simulink model "RC3_ECM"  (R2025a)
settings: Solver=VariableStepAuto  StartTime=0.0  StopTime=length(Current)  RelTol=1e-3
values from neighbouring files (symbols this model uses):
  C1_est = [C1_est(1); C1_est]    [RC3_Parameter_Extract.m]
  C2_est = [C2_est(1); C2_est]    [RC3_Parameter_Extract.m]
  C3_est = [C3_est(1); C3_est]    [RC3_Parameter_Extract.m]
  OCV_fit = flipud(OCV_fit)    [RC3_Parameter_Extract.m]    (also in RC3_Parameter_Tuning.m)
  R0_est = [R0_est(1); R0_est]    [RC3_Parameter_Extract.m]
  R1_est = [R1_est(1); R1_est]    [RC3_Parameter_Extract.m]    (also in RC3_Parameter_Tuning.m = R1_est/10)
  R2_est = [R0_est(1); R2_est]    [RC3_Parameter_Extract.m]
  R3_est = [R3_est(1); R3_est]    [RC3_Parameter_Extract.m]
  SOC_OCV = [0:0.05:1]'    [RC3_Parameter_Extract.m]    (also in RC3_Parameter_Tuning.m)
  SOC_RC = [0:0.05:1]'    [RC3_Parameter_Extract.m]    (also in RC3_Parameter_Tuning.m = [0.05:0.05:1]')
undefined symbols (not defined in the file or in its folder): OCV, Ri, SOC
settings Model: Creator=Administrator  LastModifiedBy=Administrator

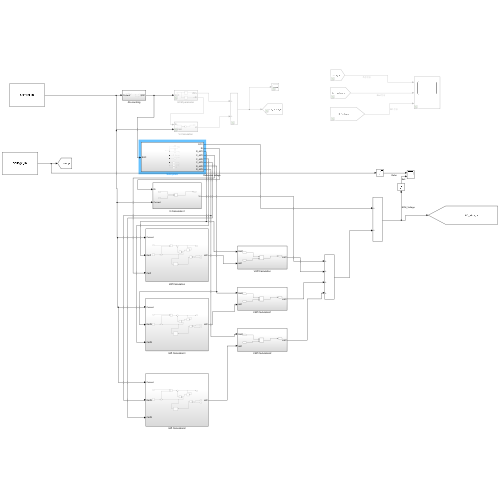
[thumbnail: Simulink's stored preview of the top-level diagram]
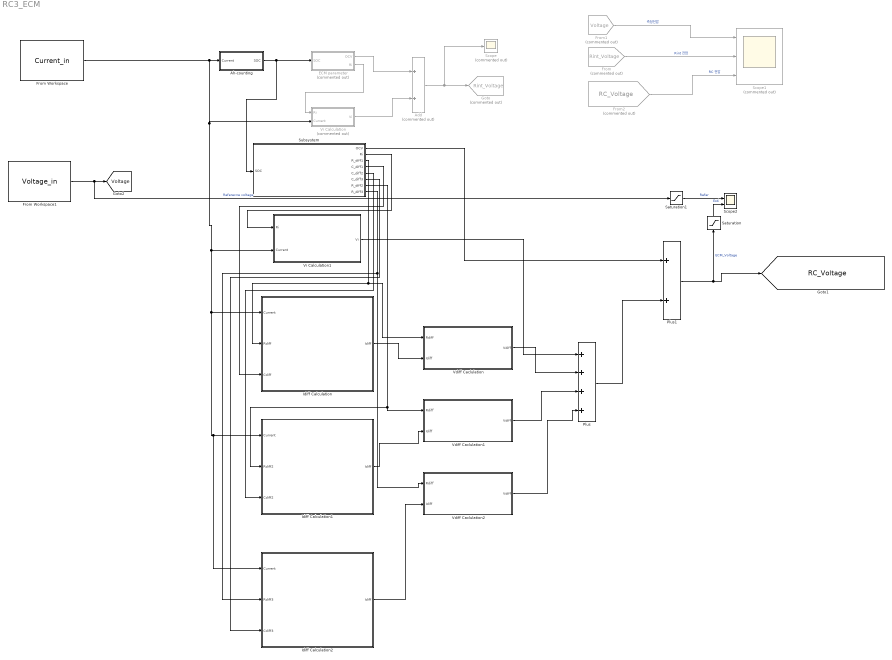
== system RC3_ECM ==
  Add : Sum  Commented=on
  Ah-counting : Subsystem
  ECM parameter : Subsystem  Commented=on
  From : From  Commented=on  GotoTag=Rint_Voltage  TagVisibility=global
  From Workspace : FromWorkspace  VariableName=Current_in  OutDataTypeStr=double  SampleTime=1
  From Workspace1 : FromWorkspace  VariableName=Voltage_in  OutDataTypeStr=double  SampleTime=1
  From1 : From  Commented=on  GotoTag=Voltage  TagVisibility=global
  From2 : From  Commented=on  GotoTag=RC_Voltage  TagVisibility=global
  Goto : Goto  Commented=on  GotoTag=Rint_Voltage  TagVisibility=global
  Idiff Calculation : Subsystem
  Idiff Calculation1 : Subsystem
  Idiff Calculation2 : Subsystem
  Plus : Sum  Inputs=++++
  Plus1 : Sum
  Saturation : Saturate  UpperLimit=4.5  LowerLimit=2.0
  Saturation1 : Saturate  UpperLimit=4.5  LowerLimit=2.0
  Scope : Scope  Commented=on
  Scope1 : Scope  Commented=on  NumInputPorts=3
      settings: ActiveDisplayYMinimum=2.8843352353917959  ActiveDisplayYMaximum=4.1440754219061109
  Scope2 : Scope  NumInputPorts=2
      settings: ActiveDisplayYMinimum=1.3491711505560249  ActiveDisplayYMaximum=4.5143277697416666  DataLoggingVariableName=ScopeVoltage
  Subsystem : Subsystem
  Vdiff Caclulation : Subsystem
  Vdiff Caclulation1 : Subsystem
  Vdiff Caclulation2 : Subsystem
  Vi Calculation : Subsystem  Commented=on
  Vi Calculation1 : Subsystem
  tag scope: RC_Voltage=global, Voltage=global
  wires:
  Ah-counting/1(SOC) -> Subsystem/1(SOC), ECM parameter/1(SOC)
  ECM parameter/1(OCV) -> Add/1
  Vi Calculation/1(Vi) -> Add/2
  Add/1 -> Scope/1, Goto/1
  ECM parameter/2(Ri) -> Vi Calculation/1(Ri)
  From Workspace/1 -> Idiff Calculation2/1(Current), Idiff Calculation1/1(Current), Idiff Calculation/1(Current), Vi Calculation1/2(Current), Vi Calculation/2(Current), Ah-counting/1(Current)
  Subsystem/2(Ri) -> Vi Calculation1/1(Ri)
  Subsystem/3(R_diff1) -> Vdiff Caclulation/1(Rdiff), Idiff Calculation/2(Rdiff)
  Subsystem/4(C_diff1) -> Idiff Calculation/3(Cdiff)
  Idiff Calculation/1(Idiff) -> Vdiff Caclulation/2(Idiff)
  Vdiff Caclulation/1(Vdiff) -> Plus/2
  Vi Calculation1/1(Vi) -> Plus/1
  Plus/1 -> Plus1/2
  Subsystem/1(OCV) -> Plus1/1
  Plus1/1 -> Saturation/1, [RC_Voltage]  "ECM_Voltage"
  From Workspace1/1 -> Saturation1/1, [Voltage]  "Referecne voltage"
  From1/1 -> Scope1/1  "측정전압"
  From/1 -> Scope1/2  "Rint 전압"
  From2/1 -> Scope1/3  "RC 전압"
  Subsystem/5(C_diff2) -> Idiff Calculation1/3(Cdiff2)
  Subsystem/6(C_diff3) -> Idiff Calculation2/3(Cdiff3)
  Subsystem/7(R_diff2) -> Vdiff Caclulation1/1(Rdiff), Idiff Calculation1/2(Rdiff2)
  Subsystem/8(R_diff3) -> Vdiff Caclulation2/1(Rdiff), Idiff Calculation2/2(Rdiff3)
  Idiff Calculation1/1(Idiff) -> Vdiff Caclulation1/2(Idiff)
  Idiff Calculation2/1(Idiff) -> Vdiff Caclulation2/2(Idiff)
  Vdiff Caclulation1/1(Vdiff) -> Plus/3
  Vdiff Caclulation2/1(Vdiff) -> Plus/4
  Saturation/1 -> Scope2/2  "Esti"
  Saturation1/1 -> Scope2/1  "Refer"

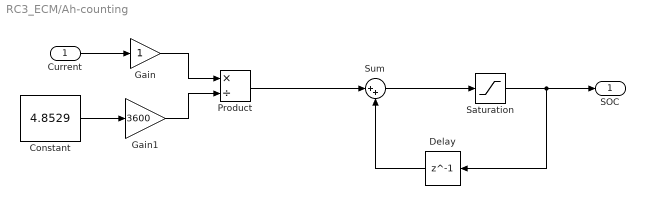
== system RC3_ECM/Ah-counting ==
  Current : Inport
  Constant : Constant  Value=4.8529
  Delay : Delay  DelayLength=1  InitialCondition=1
  Gain : Gain
  Gain1 : Gain  Gain=3600
  Product : Product  Inputs=*/
  Saturation : Saturate  UpperLimit=1  LowerLimit=0
  Sum : Sum  Inputs=|++
  SOC : Outport
  wires:
  Current/1 -> Gain/1
  Constant/1 -> Gain1/1
  Gain/1 -> Product/1
  Gain1/1 -> Product/2
  Product/1 -> Sum/1
  Sum/1 -> Saturation/1
  Saturation/1 -> Delay/1, SOC/1
  Delay/1 -> Sum/2

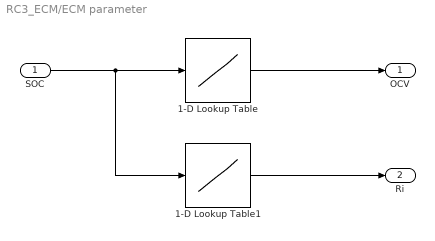
== system RC3_ECM/ECM parameter ==
  SOC : Inport
  1-D Lookup Table : Lookup_n-D  NumberOfTableDimensions=1  BreakpointsForDimension1=SOC(:,1);  Table=OCV(:,1);  InternalRulePriority=Speed  RndMeth=Simplest
  1-D Lookup Table1 : Lookup_n-D  NumberOfTableDimensions=1  BreakpointsForDimension1=SOC(:,1);  Table=Ri(:,1);  InternalRulePriority=Speed  RndMeth=Simplest
  OCV : Outport
  Ri : Outport  Port=2
  wires:
  SOC/1 -> 1-D Lookup Table1/1, 1-D Lookup Table/1
  1-D Lookup Table/1 -> OCV/1
  1-D Lookup Table1/1 -> Ri/1

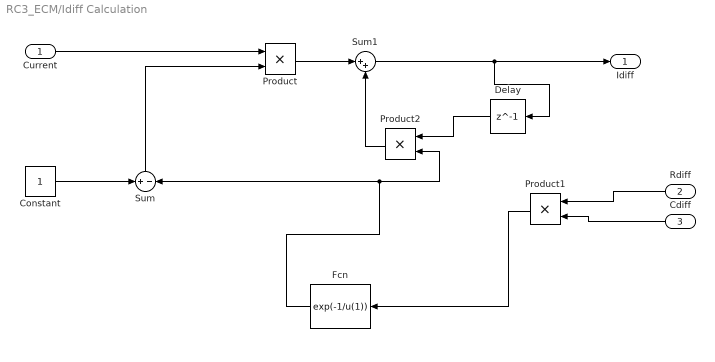
== system RC3_ECM/Idiff Calculation ==
  Current : Inport
  Rdiff : Inport  Port=2
  Cdiff : Inport  Port=3
  Constant : Constant
  Delay : Delay  DelayLength=1
  Fcn : Fcn  Expr=exp(-1/u(1))
  Product : Product
  Product1 : Product
  Product2 : Product
  Sum : Sum  Inputs=+|-
  Sum1 : Sum  Inputs=|++
  Idiff : Outport
  wires:
  Constant/1 -> Sum/1
  Current/1 -> Product/1
  Sum/1 -> Product/2
  Fcn/1 -> Sum/2, Product2/2
  Product1/1 -> Fcn/1
  Rdiff/1 -> Product1/1
  Cdiff/1 -> Product1/2
  Product2/1 -> Sum1/2
  Product/1 -> Sum1/1
  Sum1/1 -> Delay/1, Idiff/1
  Delay/1 -> Product2/1

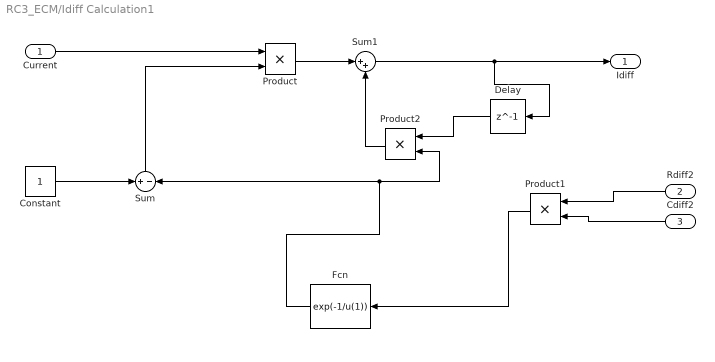
== system RC3_ECM/Idiff Calculation1 ==
  Current : Inport
  Rdiff2 : Inport  Port=2
  Cdiff2 : Inport  Port=3
  Constant : Constant
  Delay : Delay  DelayLength=1
  Fcn : Fcn  Expr=exp(-1/u(1))
  Product : Product
  Product1 : Product
  Product2 : Product
  Sum : Sum  Inputs=+|-
  Sum1 : Sum  Inputs=|++
  Idiff : Outport
  wires:
  Constant/1 -> Sum/1
  Current/1 -> Product/1
  Sum/1 -> Product/2
  Fcn/1 -> Sum/2, Product2/2
  Product1/1 -> Fcn/1
  Rdiff2/1 -> Product1/1
  Cdiff2/1 -> Product1/2
  Product2/1 -> Sum1/2
  Product/1 -> Sum1/1
  Sum1/1 -> Delay/1, Idiff/1
  Delay/1 -> Product2/1

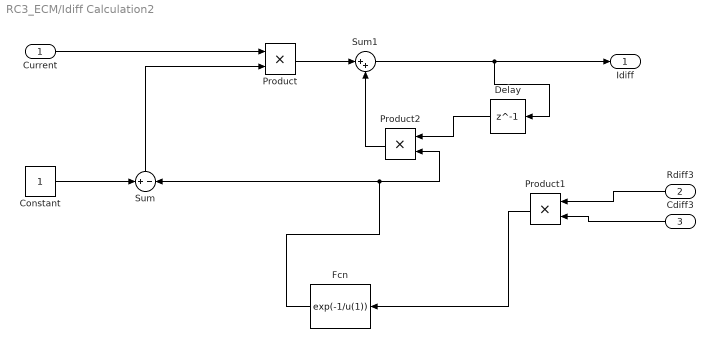
== system RC3_ECM/Idiff Calculation2 ==
  Current : Inport
  Rdiff3 : Inport  Port=2
  Cdiff3 : Inport  Port=3
  Constant : Constant
  Delay : Delay  DelayLength=1
  Fcn : Fcn  Expr=exp(-1/u(1))
  Product : Product
  Product1 : Product
  Product2 : Product
  Sum : Sum  Inputs=+|-
  Sum1 : Sum  Inputs=|++
  Idiff : Outport
  wires:
  Constant/1 -> Sum/1
  Current/1 -> Product/1
  Sum/1 -> Product/2
  Fcn/1 -> Sum/2, Product2/2
  Product1/1 -> Fcn/1
  Rdiff3/1 -> Product1/1
  Cdiff3/1 -> Product1/2
  Product2/1 -> Sum1/2
  Product/1 -> Sum1/1
  Sum1/1 -> Delay/1, Idiff/1
  Delay/1 -> Product2/1

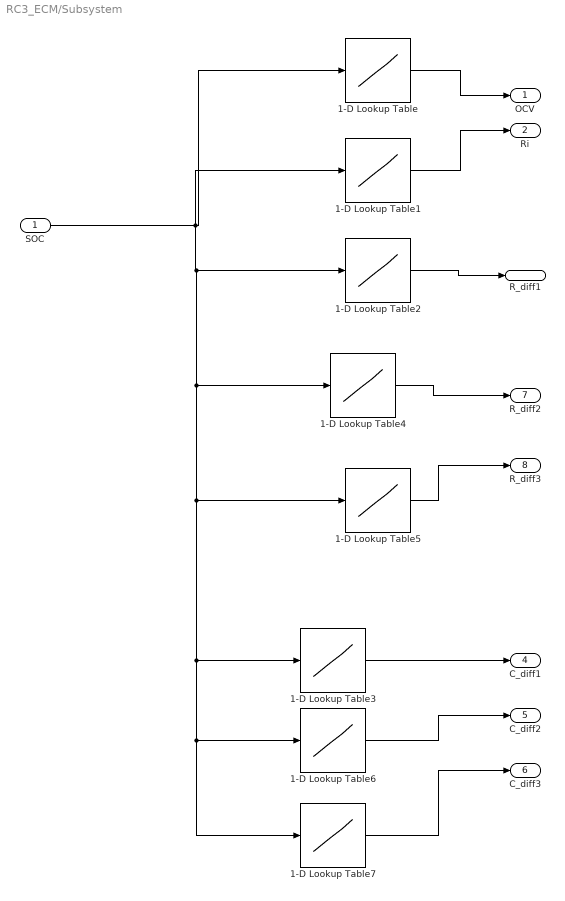
== system RC3_ECM/Subsystem ==
  SOC : Inport
  1-D Lookup Table : Lookup_n-D  NumberOfTableDimensions=1  BreakpointsForDimension1=SOC_OCV  Table=OCV_fit  InternalRulePriority=Speed  RndMeth=Simplest
  1-D Lookup Table1 : Lookup_n-D  NumberOfTableDimensions=1  BreakpointsForDimension1=SOC_RC  Table=R0_est  InternalRulePriority=Speed  RndMeth=Simplest
  1-D Lookup Table2 : Lookup_n-D  NumberOfTableDimensions=1  BreakpointsForDimension1=SOC_RC  Table=R1_est  InternalRulePriority=Speed  RndMeth=Simplest
  1-D Lookup Table3 : Lookup_n-D  NumberOfTableDimensions=1  BreakpointsForDimension1=SOC_RC  Table=C1_est  InternalRulePriority=Speed  RndMeth=Simplest
  1-D Lookup Table4 : Lookup_n-D  NumberOfTableDimensions=1  BreakpointsForDimension1=SOC_RC  Table=R2_est  InternalRulePriority=Speed  RndMeth=Simplest
  1-D Lookup Table5 : Lookup_n-D  NumberOfTableDimensions=1  BreakpointsForDimension1=SOC_RC  Table=R3_est  InternalRulePriority=Speed  RndMeth=Simplest
  1-D Lookup Table6 : Lookup_n-D  NumberOfTableDimensions=1  BreakpointsForDimension1=SOC_RC  Table=C2_est  InternalRulePriority=Speed  RndMeth=Simplest
  1-D Lookup Table7 : Lookup_n-D  NumberOfTableDimensions=1  BreakpointsForDimension1=SOC_RC  Table=C3_est  InternalRulePriority=Speed  RndMeth=Simplest
  OCV : Outport
  Ri : Outport  Port=2
  R_diff1 : Outport  Port=3
  C_diff1 : Outport  Port=4
  C_diff2 : Outport  Port=5
  C_diff3 : Outport  Port=6
  R_diff2 : Outport  Port=7
  R_diff3 : Outport  Port=8
  wires:
  1-D Lookup Table/1 -> OCV/1
  1-D Lookup Table1/1 -> Ri/1
  1-D Lookup Table2/1 -> R_diff1/1
  1-D Lookup Table3/1 -> C_diff1/1
  SOC/1 -> 1-D Lookup Table4/1, 1-D Lookup Table7/1, 1-D Lookup Table6/1, 1-D Lookup Table3/1, 1-D Lookup Table5/1, 1-D Lookup Table2/1, 1-D Lookup Table1/1, 1-D Lookup Table/1
  1-D Lookup Table4/1 -> R_diff2/1
  1-D Lookup Table5/1 -> R_diff3/1
  1-D Lookup Table6/1 -> C_diff2/1
  1-D Lookup Table7/1 -> C_diff3/1

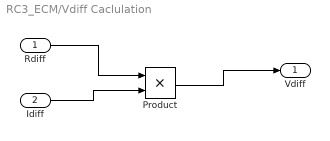
== system RC3_ECM/Vdiff Caclulation ==
  Rdiff : Inport
  Idiff : Inport  Port=2
  Product : Product
  Vdiff : Outport
  wires:
  Idiff/1 -> Product/2
  Rdiff/1 -> Product/1
  Product/1 -> Vdiff/1

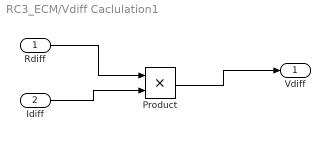
== system RC3_ECM/Vdiff Caclulation1 ==
  Rdiff : Inport
  Idiff : Inport  Port=2
  Product : Product
  Vdiff : Outport
  wires:
  Idiff/1 -> Product/2
  Rdiff/1 -> Product/1
  Product/1 -> Vdiff/1

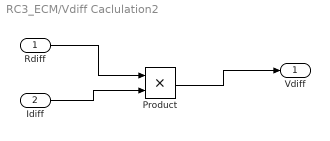
== system RC3_ECM/Vdiff Caclulation2 ==
  Rdiff : Inport
  Idiff : Inport  Port=2
  Product : Product
  Vdiff : Outport
  wires:
  Idiff/1 -> Product/2
  Rdiff/1 -> Product/1
  Product/1 -> Vdiff/1

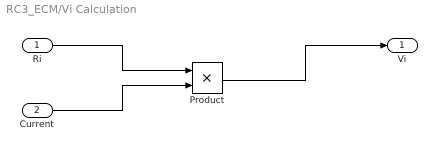
== system RC3_ECM/Vi Calculation ==
  Ri : Inport
  Current : Inport  Port=2
  Product : Product
  Vi : Outport
  wires:
  Current/1 -> Product/2
  Product/1 -> Vi/1
  Ri/1 -> Product/1

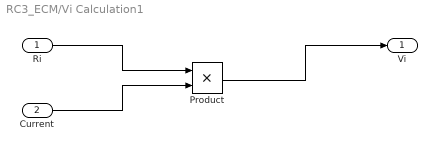
== system RC3_ECM/Vi Calculation1 ==
  Ri : Inport
  Current : Inport  Port=2
  Product : Product
  Vi : Outport
  wires:
  Current/1 -> Product/2
  Product/1 -> Vi/1
  Ri/1 -> Product/1
